simulink model "ptest3sim21"  (Simulink 8.6)
settings: Solver=FixedStepDiscrete  SolverMode=SingleTasking  StartTime=0.0  StopTime=999999  MaxStep=10  RelTol=1e-3  AbsTol=1e-6
settings Model: Creator=The MathWorks, Inc.  LastModifiedBy=98915  ExtModeTrigMode=oneshot  ExtModeArmWhenConnect=off
settings DataIOCC: LimitDataPoints=off  SignalLoggingSaveFormat=Dataset  SaveOutput=off  SaveTime=off
settings OptimizationCC: BooleanDataType=off  ExpressionDepthLimit=128  InitFltsAndDblsToZero=on
settings DebuggingCC: SaveWithParameterizedLinksMsg=none  SignalResolutionControl=TryResolveAllWithWarning  SolverPrmCheckMsg=none  MultiTaskDSMMsg=warning  MultiTaskCondExecSysMsg=none  FcnCallInpInsideContextMsg=UseLocalSettings  StateNameClashWarn=none  StrictBusMsg=None
settings HardwareCC: TargetUnknown=on
settings RTWCC: TemplateMakefile=grt_vc.tmf
settings GRTTargetCC: TargetFcnLib=ansi_tfl_tmw.mat  GeneratePreprocessorConditionals=Use local settings

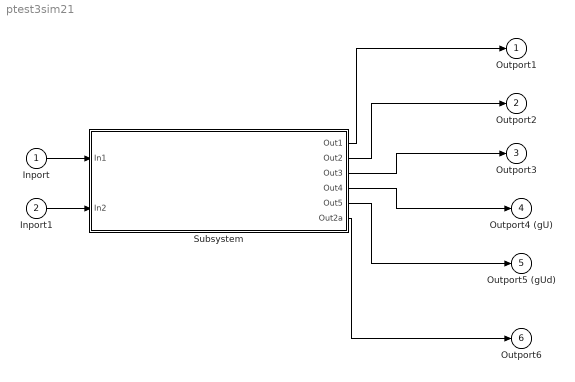
== system ptest3sim21 ==
  Inport : Inport  PortDimensions=1
  Inport1 : Inport  Port=2  PortDimensions=1
  Subsystem : Subsystem  mask{yd_init1=[], y_init1=[], ud_init1=[], u_init1=[], mint1=217.62128892307953, maxt1=34.372117523742894, minp1=-14.518123641385754, maxp1=34.372117523742894, Ts1=0.05, S11=30, Nu1=2, Normalize1=0, Nj1=8, Ni1=3, LW2_11=[-26.064437811822213 22.382889355042366 22.398837452917832 -0.038286916694043924 1.216688905180568 0.10267800941528266 -31.001649977902009 22.809795495362049 0.14942990031167722 0.048217737772188428 -4.4707432115359147 0.12178330692895029 -0.23851607275022915 -23.921580806620806 0.054556286879472386 -24.423700290603563 0.70273727827187649 -22.882781864161863 -24.604415673380409 -0.081830133233886743 -0.13387227258563716 -1.0474484701964166 -0.016841195793368118 0.11673448004303272 0.22617275989991151 25.430599242235367 22.099207513017429 -2.8763089810507201 -0.56899532933082742 0.30349310587430406], LW1_21=[0.14502232133705253 -0.19818602514849301 -0.60030350491395079 -0.1091436710422941 0.33409735053318945 -0.22419571803249635 -0.11973734213668785 0.17770764249420579;0.61880869696550134 0.97723668947232223 1.3461112999321452 0.3542669376814257 -0.55884694662707912 -0.28939105831102441 -0.68790748729887186 -0.33182701878380871;-0.26934359396580165 -0.094325885979179278 -0.0051102057497130968 0.65645318710181122 -0.43125476840555776 0.95812084203300774 0.13802281101576963 0.025946861741987223;-8.7196630145784848 6.8832507745514659 -0.26746057163670217 1.6903423388513836 3.1068326405173576 -13.658263649124519 6.3432430899147514 5.1557368296910964;-0.42053330941632955 0.0021066596747489549 2.3804057933097043 -0.66379186998163353 -2.2639798510471443 -2.1967847104136267 -0.8763419273661075 2.1150437956429156;-7.1419732168053276 6.531169454969092 2.7215070785300126 7.0971881132216801 -3.5746092990403722 -6.5025240568661253 -6.6290198132326461 6.8568101700956525;-0.015771842955708899 0.0057460854063624087 -0.00056353334053432336 0.00021011981240546708 -7.4544898266139608e-05 0.00039588102987094778 0.00044677216599032772 -0.0014763192468849311;0.31151126507962201 0.11936889656995812 0.067520964291386834 0.12451305995171068 -0.036455595088563678 -0.27775588229622139 -0.35117788310761511 0.20728982648327363;11.390624155429196 -8.3433809517666262 -9.4147211666194917 -4.8690895934680718 10.081396381472576 6.0836080054306887 -1.5840948822947798 -3.2969620561875552;1.0838166192685366 2.8302531028433888 6.0145929419319568 7.1158034515286479 9.6848381769370597 -4.7393408643914956 -16.78957164310528 -4.9485693068314962;-1.2072042547676116 -0.10007996802061325 -0.56957359064428426 0.31160078810101088 -0.52907645533917813 0.54983749296665951 -0.13793506464915217 -0.7486731666214963;0.49642374282030055 -0.91929128492921641 -3.9060463084663337 7.2702803268945964 7.3561279992136575 -6.7738310516435716 -1.0602552755938028 -2.4638781476749152;-0.93518454404494655 5.2998976823039143 3.8608812498302982 -5.0894727406121811 -3.4015910704902041 0.86539048744327884 0.39814684093945646 3.3621968909144693;-0.0035735280319696555 -0.10656868580625431 -0.061320877011787484 -0.035511896314988869 0.0041861499133045918 -0.015968778853224376 -0.047093240620693602 -0.064798701154283239;-8.2722783163792819 6.3466203448402334 9.8759249225987595 0.76387799542218671 -6.8167353900920613 -0.77527271379467255 0.81361460958365017 -3.0326228793873296;0.37380922340158035 0.6391160962361726 -1.2495932575943429 -0.28017027281391477 -0.74666397338505752 0.065941275603083715 0.69166332882506598 0.20136822412624111;2.6115793379678371 -6.0681600126871462 4.7445282811131637 -3.5610352160654468 -10.359909014176985 10.563424520127153 -9.0756344807167046 16.518703424325352;-0.70234986199369964 -0.17469610726357687 -0.03001669111107063 0.02612133762570161 0.082789827161885182 -0.0006553685984739782 0.28277301528104837 0.21236907072855862;-0.003946231444981383 -0.64512381160267984 -1.7987939159474886 0.99773115006692348 0.24897143993074494 -0.5115453193903271 -0.048266160438610116 1.2190161110380973;6.8673264325130532 7.3803565449334778 -9.3143920545849337 -7.7132136285015722 -0.038113443475049379 -0.19907892662547941 3.1378648399070221 0.38685604142055852;-10.080746690315406 1.586722263572262 1.1906230862174914 1.2601665584162989 -4.8438413621869447 -2.3124231961994854 21.692379716674314 -9.556199690855669;0.50394263177350407 13.666229500118867 -6.4353963093274356 2.8787469553955596 -3.7661310538645001 0.065584133519514198 -4.7658927478393345 1.3776799184387216;-25.209345319364061 -4.0686774170865609 8.6463104242327997 -3.7201723905081718 -0.65310481926140851 10.099887870222826 4.4989934760756434 9.1387531060497924;0.3525198504373101 0.19932470222582813 -2.0493336024776427 -0.3271272328144369 0.5052560341723944 -3.3039844970379195 3.8047824205524825 -3.5061638492871174;-1.9580626778247048 -3.1549493778988245 -8.4717854780401893 -0.85467953969785948 2.9569972800286322 2.2831828826620972 ...(+840 chars)], IW_gU1=[0.033749633509924319 0.51953797110680611 0.023953451058919214;-1.0570051190545673 -1.1537719859033251 0.42725864185800633;0.78198964403097426 -1.9244427859818585 -1.1072794700998263;-2.665630567437741 4.477362363430867 -7.3543001126906802;0.21961341017723846 0.54708393700106972 -0.26136462634935154;4.8729663671470229 1.3701805335023274 -1.0133600095268858;-0.020104489318732578 0.010062701534381654 -0.0039861656524516394;0.13212814395498115 0.88938303327521406 0.70243984219654032;-4.7645188512536549 3.3805095101858416 -1.0232751022757849;7.5371264222675549 -12.790033145066447 4.2322004394291248;-0.46616123477808313 -0.52800676314474115 0.8378056528735468;-13.531196625565929 9.0933120302301464 6.3144783944710534;-9.2656430427380982 -11.822209180334529 -11.079518571007783;-3.4594199678477516e-06 -0.024067454126836117 -0.053008941256448602;-18.968530056782342 -10.000225011921206 -3.162982825532243;0.31016269407956709 -0.33899020830424847 -0.076532678861312126;8.5236807005538946 5.793482018308266 0.2267443105300363;-0.98798745799044374 -1.0407776006619636 0.043771841805682034;-1.4186006521322074 1.5182006130106442 -0.27506256155117775;-0.83263801153775019 2.1589660973629616 -7.3848566431678586;10.546585044494808 11.239237542296129 -0.086595538531225091;1.1144254437189585 -8.6727039498850633 -7.9974962312798965;4.7891727215344666 -5.5975119529414235 9.7078941580829721;13.658156109610113 14.054243379505479 13.83709294556418;16.70226268039049 -8.19270321836993 -9.798271605925704;0.13904179904099778 0.77678213857190559 1.3944541255894785;1.4499358486282008 -0.051626218254679161 -0.84425652617503177;-14.699896211239166 13.082109346033086 10.652415472508936;-1.6396349693196193 1.3329230717599549 0.78660485907763611;-0.58060303719033945 1.7004396167783182 -13.0281679262245], IW1=[0.033749633509924319 0.51953797110680611 0.023953451058919214;-1.0570051190545673 -1.1537719859033251 0.42725864185800633;0.78198964403097426 -1.9244427859818585 -1.1072794700998263;-2.665630567437741 4.477362363430867 -7.3543001126906802;0.21961341017723846 0.54708393700106972 -0.26136462634935154;4.8729663671470229 1.3701805335023274 -1.0133600095268858;-0.020104489318732578 0.010062701534381654 -0.0039861656524516394;0.13212814395498115 0.88938303327521406 0.70243984219654032;-4.7645188512536549 3.3805095101858416 -1.0232751022757849;7.5371264222675549 -12.790033145066447 4.2322004394291248;-0.46616123477808313 -0.52800676314474115 0.8378056528735468;-13.531196625565929 9.0933120302301464 6.3144783944710534;-9.2656430427380982 -11.822209180334529 -11.079518571007783;-3.4594199678477516e-06 -0.024067454126836117 -0.053008941256448602;-18.968530056782342 -10.000225011921206 -3.162982825532243;0.31016269407956709 -0.33899020830424847 -0.076532678861312126;8.5236807005538946 5.793482018308266 0.2267443105300363;-0.98798745799044374 -1.0407776006619636 0.043771841805682034;-1.4186006521322074 1.5182006130106442 -0.27506256155117775;-0.83263801153775019 2.1589660973629616 -7.3848566431678586;10.546585044494808 11.239237542296129 -0.086595538531225091;1.1144254437189585 -8.6727039498850633 -7.9974962312798965;4.7891727215344666 -5.5975119529414235 9.7078941580829721;13.658156109610113 14.054243379505479 13.83709294556418;16.70226268039049 -8.19270321836993 -9.798271605925704;0.13904179904099778 0.77678213857190559 1.3944541255894785;1.4499358486282008 -0.051626218254679161 -0.84425652617503177;-14.699896211239166 13.082109346033086 10.652415472508936;-1.6396349693196193 1.3329230717599549 0.78660485907763611;-0.58060303719033945 1.7004396167783182 -13.0281679262245], B21=24.992136850997451, B11=[-36.093687166784058;-12.305889740475774;-5.3023355649171329;-12.182040660818414;10.135270477537007;8.0430063124967486;3.0174318673985403;29.621858949022169;-0.48454974365016329;-32.040207569052725;-19.070457729234576;20.548211928919049;-2.0183656641746404;-8.1912048609880159;40.791767675235391;4.6706071066423558;9.7388139484696374;-41.138203994054322;-8.2477628443093263;25.890733055108694;-25.299908828489205;-45.374295607353503;34.392721015628311;0.74592894079050842;-15.073682539786347;-30.718114798670658;25.564327668539196;-23.56231663956774;29.489094041256738;-8.6827696859839438]}
  Outport1 : Outport
  Outport2 : Outport  Port=2
  Outport3 : Outport  Port=3
  Outport4 (gU) : Outport  Port=4
  Outport5 (gUd) : Outport  Port=5
  Outport6 : Outport  Port=6
  wires:
  Subsystem/2(Out2) -> Outport2/1
  Subsystem/1(Out1) -> Outport1/1
  Subsystem/3(Out3) -> Outport3/1
  Inport1/1 -> Subsystem/2(In2)
  Subsystem/5(Out5) -> Outport5 (gUd)/1
  Inport/1 -> Subsystem/1(In1)
  Subsystem/4(Out4) -> Outport4 (gU)/1
  Subsystem/6(Out2a) -> Outport6/1

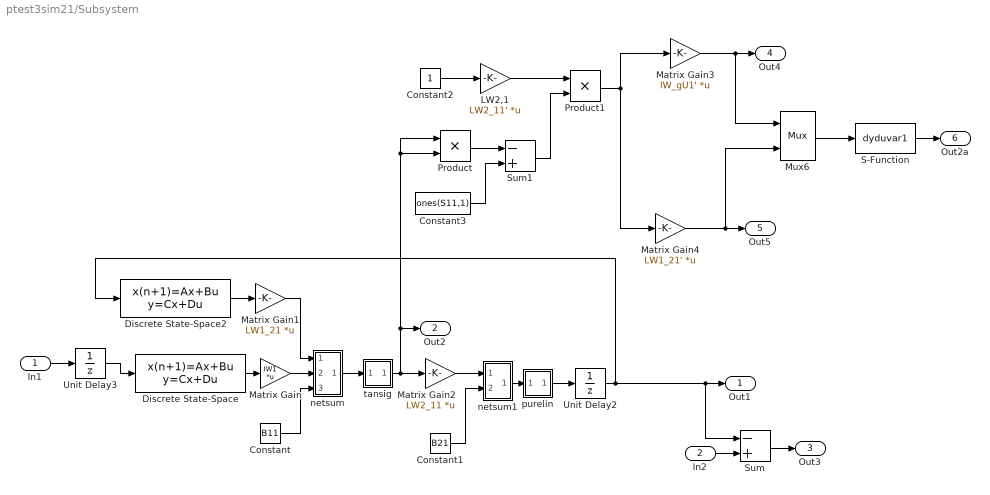
== system ptest3sim21/Subsystem ==
  In1 : Inport
  In2 : Inport  Port=2
  Constant : Constant  Value=B11
  Constant1 : Constant  Value=B21
  Constant2 : Constant
  Constant3 : Constant  Value=ones(S11,1)
  Discrete State-Space : DiscreteStateSpace  A=[0 zeros(1,Ni1-2);eye(Ni1-2,Ni1-1)]  B=[zeros(double(Ni1==1));eye(Ni1-1,1)]  C=[0 zeros(1,Ni1-2);eye(Ni1-1,Ni1-1)]  D=eye(Ni1,1)  X0=ud_init1  SampleTime=Ts1
  Discrete State-Space2 : DiscreteStateSpace  A=[0 zeros(1,Nj1-2);eye(Nj1-2,Nj1-1)]  B=[zeros(double(Nj1==1));eye(Nj1-1,1)]  C=[0 zeros(1,Nj1-2);eye(Nj1-1,Nj1-1)]  D=eye(Nj1,1)  X0=yd_init1  SampleTime=Ts1
  LW2,1 : Gain  Gain=LW2_11'  Multiplication=Matrix(K*u)  SaturateOnIntegerOverflow=on  OutDataTypeStr=Inherit: Same as input  ParamDataTypeStr=Inherit: Same as input
  Matrix Gain : Gain  Gain=IW1  Multiplication=Matrix(K*u)  SaturateOnIntegerOverflow=on  OutDataTypeStr=Inherit: Same as input  ParamDataTypeStr=Inherit: Same as input
  Matrix Gain1 : Gain  Gain=LW1_21  Multiplication=Matrix(K*u)  SaturateOnIntegerOverflow=on  OutDataTypeStr=Inherit: Same as input  ParamDataTypeStr=Inherit: Same as input
  Matrix Gain2 : Gain  Gain=LW2_11  Multiplication=Matrix(K*u)  SaturateOnIntegerOverflow=on  OutDataTypeStr=Inherit: Same as input  ParamDataTypeStr=Inherit: Same as input
  Matrix Gain3 : Gain  Gain=IW_gU1'  Multiplication=Matrix(K*u)  SaturateOnIntegerOverflow=on  OutDataTypeStr=Inherit: Same as input  ParamDataTypeStr=Inherit: Same as input
  Matrix Gain4 : Gain  Gain=LW1_21'  Multiplication=Matrix(K*u)  SaturateOnIntegerOverflow=on  OutDataTypeStr=Inherit: Same as input  ParamDataTypeStr=Inherit: Same as input
  Mux6 : Mux  Inputs=2
  Product : Product  SaturateOnIntegerOverflow=on  RndMeth=Zero  InputSameDT=on  OutDataTypeStr=Inherit: Same as first input
  Product1 : Product  SaturateOnIntegerOverflow=on  RndMeth=Zero  InputSameDT=on  OutDataTypeStr=Inherit: Same as first input
  S-Function : S-Function  FunctionName=dyduvar1  Parameters=Nu1,Ni1,Nj1,Ts1,minp1,maxp1,mint1,maxt1,Normalize1  SFunctionDeploymentMode=off  EnableBusSupport=off
  Sum : Sum  Inputs=-+  SaturateOnIntegerOverflow=on  InputSameDT=on  OutDataTypeStr=Inherit: Same as first input
  Sum1 : Sum  Inputs=-+  SaturateOnIntegerOverflow=on  InputSameDT=on  OutDataTypeStr=Inherit: Same as first input
  Unit Delay2 : UnitDelay  InitialCondition=y_init1  SampleTime=Ts1
  Unit Delay3 : UnitDelay  InitialCondition=u_init1  SampleTime=Ts1
  netsum : Subsystem
      mask Display: disp('+')
  netsum1 : Subsystem
      mask Display: disp('+')
  purelin : Subsystem
      mask Display: plot([-1 1],[0 0],[-1 1],[-1 1])
  tansig : Subsystem
      mask Display: plot([-1 1],[0 0],[-1 -.9 -.8 -.7 -.6 -.5 -.4 -.3 -.2 -.1 0 .1 .2 .3 .4 .5 .6 .7 .8 .9 1],2./(1+exp(-8*[-1 -.9 -.8 -.7 -.6 -.5 -.4 -.3 -.2 -.1 0 .1 .2 .3 .4 .5 .6 .7 .8 .9 1]))-1)
  Out1 : Outport
  Out2 : Outport  Port=2
  Out3 : Outport  Port=3
  Out4 : Outport  Port=4
  Out5 : Outport  Port=5
  Out2a : Outport  Port=6
  wires:
  LW2,1/1 -> Product1/1
  Product1/1 -> Matrix Gain4/1, Matrix Gain3/1
  Constant2/1 -> LW2,1/1
  Product/1 -> Sum1/1
  Constant3/1 -> Sum1/2
  Sum1/1 -> Product1/2
  netsum1/1(Out1) -> purelin/1(n)
  Constant1/1 -> netsum1/2(In2)
  Matrix Gain2/1 -> netsum1/1(In1)
  Constant/1 -> netsum/3(In3)
  Matrix Gain1/1 -> netsum/1(In1)
  Discrete State-Space2/1 -> Matrix Gain1/1
  Matrix Gain/1 -> netsum/2(In2)
  tansig/1(a) -> Product/1, Product/2, Out2/1, Matrix Gain2/1
  purelin/1(a) -> Unit Delay2/1
  Unit Delay2/1 -> Discrete State-Space2/1, Sum/1, Out1/1
  Discrete State-Space/1 -> Matrix Gain/1
  Matrix Gain4/1 -> Mux6/2, Out5/1
  Mux6/1 -> S-Function/1
  Unit Delay3/1 -> Discrete State-Space/1
  Matrix Gain3/1 -> Mux6/1, Out4/1
  S-Function/1 -> Out2a/1
  In1/1 -> Unit Delay3/1
  Sum/1 -> Out3/1
  In2/1 -> Sum/2
  netsum/1(Out1) -> tansig/1(n)

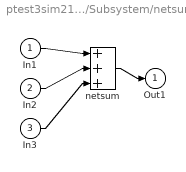
== system ptest3sim21/Subsystem/netsum ==
  In1 : Inport
  In2 : Inport  Port=2
  In3 : Inport  Port=3
  netsum : Sum  Inputs=3  SaturateOnIntegerOverflow=on  InputSameDT=on  OutDataTypeStr=Inherit: Same as first input
  Out1 : Outport
  wires:
  In1/1 -> netsum/1
  In2/1 -> netsum/2
  In3/1 -> netsum/3
  netsum/1 -> Out1/1

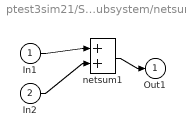
== system ptest3sim21/Subsystem/netsum1 ==
  In1 : Inport
  In2 : Inport  Port=2
  netsum1 : Sum  Inputs=2  SaturateOnIntegerOverflow=on  InputSameDT=on  OutDataTypeStr=Inherit: Same as first input
  Out1 : Outport
  wires:
  In1/1 -> netsum1/1
  In2/1 -> netsum1/2
  netsum1/1 -> Out1/1

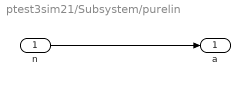
== system ptest3sim21/Subsystem/purelin ==
  n : Inport
  a : Outport
  wires:
  n/1 -> a/1

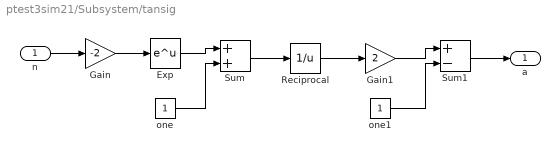
== system ptest3sim21/Subsystem/tansig ==
  n : Inport
  Exp : Math  SaturateOnIntegerOverflow=on
  Gain : Gain  Gain=-2  SaturateOnIntegerOverflow=on  OutDataTypeStr=Inherit: Same as input  ParamDataTypeStr=Inherit: Same as input
  Gain1 : Gain  Gain=2  SaturateOnIntegerOverflow=on  OutDataTypeStr=Inherit: Same as input  ParamDataTypeStr=Inherit: Same as input
  Reciprocal : Math  Operator=reciprocal  SaturateOnIntegerOverflow=on
  Sum : Sum  SaturateOnIntegerOverflow=on  InputSameDT=on  OutDataTypeStr=Inherit: Same as first input
  Sum1 : Sum  Inputs=+-  SaturateOnIntegerOverflow=on  InputSameDT=on  OutDataTypeStr=Inherit: Same as first input
  one : Constant
  one1 : Constant
  a : Outport
  wires:
  n/1 -> Gain/1
  Gain/1 -> Exp/1
  Exp/1 -> Sum/1
  one/1 -> Sum/2
  Sum/1 -> Reciprocal/1
  Reciprocal/1 -> Gain1/1
  Gain1/1 -> Sum1/1
  one1/1 -> Sum1/2
  Sum1/1 -> a/1
